simulink model "SMC"  (R2024b)
settings: Solver=FixedStepAuto  StartTime=0.0  StopTime=10  FixedStep=0.00001  MinStep=1e-6  RelTol=1e-9
InitFcn:
  | addpath('./../Robot Description/Robot Data Package/meshes/visual/')
  | addpath('./../Dynamics and Kinematics/')
  | 
  | % Controller Design
  | Design;
values from neighbouring files (symbols this model uses):
  Eta = 50000    [Design.m]
  Lambda = 50000    [Design.m]
  qInitDM = [rand(7, 1); zeros(7, 1)]    [Design.m]
settings Model: Creator=Banaan  LastModifiedBy=Banaan

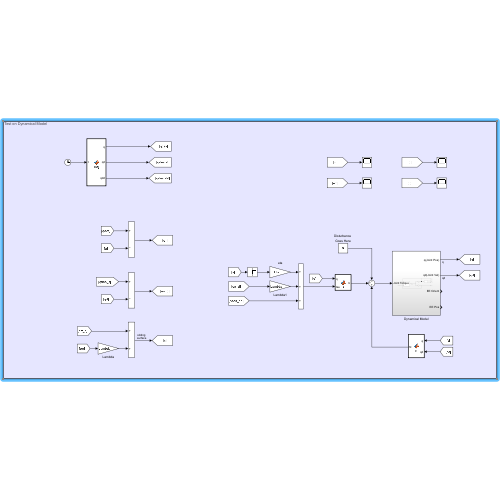
[thumbnail: Simulink's stored preview of the top-level diagram]
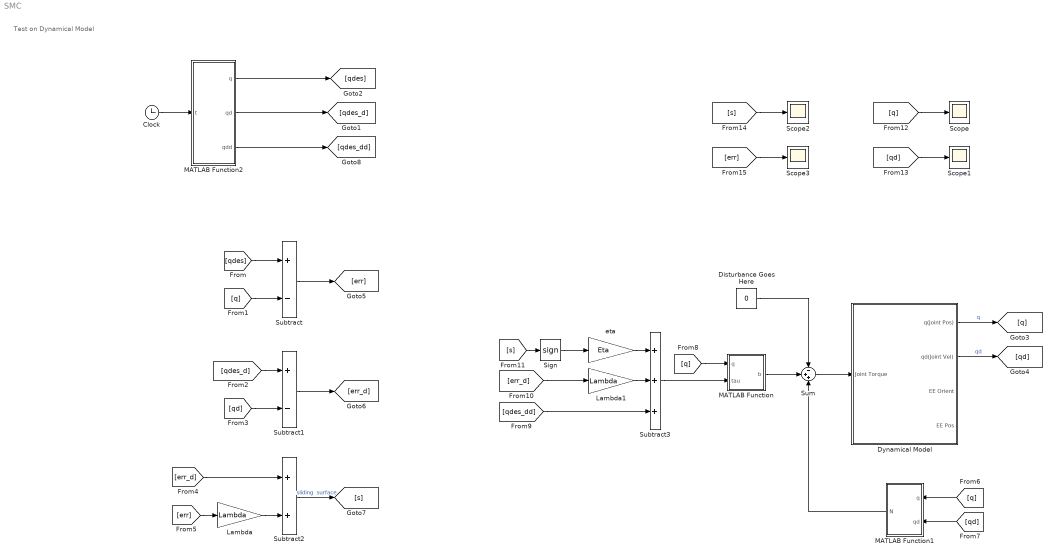
== system SMC ==
  note: Test on Dynamical Model
  Clock : Clock
  Disturbance Goes Here : Constant  Value=0
  Dynamical Model : Subsystem
  Lambda : Gain  Gain=Lambda
  Lambda1 : Gain  Gain=Lambda
  MATLAB Function : MATLAB Function  TreatAsAtomicUnit=on
  MATLAB Function1 : MATLAB Function  TreatAsAtomicUnit=on
  MATLAB Function2 : MATLAB Function  TreatAsAtomicUnit=on
  Scope{,1..3} (4 alike) : Scope
  Sign : Signum  ZeroCross=off
  Subtract : Sum  Inputs=+-
  Subtract1 : Sum  Inputs=+-
  Subtract2 : Sum
  Subtract3 : Sum  Inputs=+++
  Sum : Sum  Inputs=-++
  eta : Gain  Gain=Eta
  wires:
  Dynamical Model/1(q(Joint Pos)) -> [q]  "q"
  Dynamical Model/2(qd(Joint Vel)) -> [qd]  "qd"
  [qdes] -> Subtract/1
  [q] -> Subtract/2
  Subtract/1 -> [err]
  Subtract1/1 -> [err_d]
  [qd] -> Subtract1/2
  [qdes_d] -> Subtract1/1
  [err_d] -> Subtract2/1
  [err] -> Lambda/1
  Subtract2/1 -> [s]  "sliding  surface"
  Lambda/1 -> Subtract2/2
  Sum/1 -> Dynamical Model/1(Joint Torque)
  Disturbance Goes Here/1 -> Sum/1
  [q] -> MATLAB Function1/1(q)
  [qd] -> MATLAB Function1/2(qd)
  MATLAB Function1/1(N) -> Sum/3
  MATLAB Function/1(b) -> Sum/2
  [q] -> MATLAB Function/1(q)
  Subtract3/1 -> MATLAB Function/2(tau)
  [qdes_dd] -> Subtract3/3
  [err_d] -> Lambda1/1
  Lambda1/1 -> Subtract3/2
  eta/1 -> Subtract3/1
  Sign/1 -> eta/1
  [s] -> Sign/1
  [q] -> Scope/1
  [qd] -> Scope1/1
  [err] -> Scope3/1
  [s] -> Scope2/1
  Clock/1 -> MATLAB Function2/1(t)
  MATLAB Function2/3(qdd) -> [qdes_dd]
  MATLAB Function2/2(qd) -> [qdes_d]
  MATLAB Function2/1(q) -> [qdes]

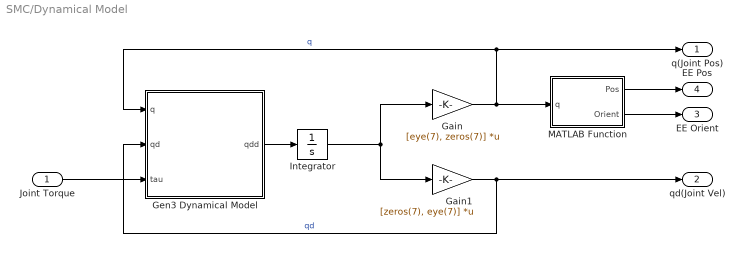
== system SMC/Dynamical Model ==
  Joint Torque : Inport
  Gain : Gain  Gain=[eye(7), zeros(7)]  Multiplication=Matrix(K*u)
  Gain1 : Gain  Gain=[zeros(7), eye(7)]  Multiplication=Matrix(K*u)
  Gen3 Dynamical Model : MATLAB Function  TreatAsAtomicUnit=on
  Integrator : Integrator  InitialCondition=qInitDM
  MATLAB Function : MATLAB Function  TreatAsAtomicUnit=on
  q(Joint Pos) : Outport
  qd(Joint Vel) : Outport  Port=2
  EE Orient : Outport  Port=3
  EE Pos : Outport  Port=4
  wires:
  Integrator/1 -> Gain/1, Gain1/1
  Gain/1 -> MATLAB Function/1(q), Gen3 Dynamical Model/1(q), q(Joint Pos)/1  "q"
  Gen3 Dynamical Model/1(qdd) -> Integrator/1
  Gain1/1 -> qd(Joint Vel)/1, Gen3 Dynamical Model/2(qd)  "qd"
  Joint Torque/1 -> Gen3 Dynamical Model/3(tau)
  MATLAB Function/1(Pos) -> EE Pos/1
  MATLAB Function/2(Orient) -> EE Orient/1

== matlab function SMC/MATLAB Function2 ==
  data: t input; q output; qd output; qdd output
function [q, qd, qdd] = Traj(t)

    q   =  ones(7, 1) * sin(t);
    qd  =  ones(7, 1) * cos(t);
    qdd = -ones(7, 1) * sin(t);

end

== matlab function SMC/Dynamical Model/MATLAB Function ==
  data: q input; Pos output; Orient output
function [Pos, Orient] = FK(q) %#codegen
    coder.extrinsic('Gen3FK');

    tmp = zeros(6, 1);
    tmp = Gen3FK(q);

    Pos    = tmp(1:3, 1);
    Orient = tmp(4:6, 1);      % Order = [Yaw - Pitch - Roll]
end

== matlab function SMC/MATLAB Function ==
  data: q input; b output; tau input
function b = B(q, tau) %#codegen
    coder.extrinsic('Gen3ODEFun_B');

    tmp = zeros(7, 7);
    tmp = Gen3ODEFun_B(q);

    b = zeros(7, 1);
    b = tmp * tau;
end

== matlab function SMC/MATLAB Function1 ==
  data: q input; N output; qd input
function N = n(q, qd) %#codegen
    coder.extrinsic('Gen3ODEFun_C');
    coder.extrinsic('Gen3ODEFun_g');

    N = zeros(7, 1);
    C = zeros(7, 7);
    g = zeros(7, 1);
    
    C = Gen3ODEFun_C(q, qd);
    g = Gen3ODEFun_g(q);
    N = C * qd + g;
end

== matlab function SMC/Dynamical Model/Gen3 Dynamical Model ==
  data: q input; qdd output; qd input; tau input
function qdd = fcn(q, qd, tau) %#codegen
    coder.extrinsic('Gen3ODEFun');

    qdd = zeros(14, 1);
    qdd = Gen3ODEFun(0, [q; qd], tau);
end
